simulink model "rosberrypi_publish_camera"  (R2018b)
settings: Solver=FixedStepAuto  StartTime=0.0  StopTime=inf  RelTol=1e-3  EnableMultiTasking=on
model workspace (MAT data in the model file):
  SL_ROS_VariableLengthArrays_MaxSizes.CommonInfo.ArrayTruncateAction = 'EmitWarning'
  SL_ROS_VariableLengthArrays_MaxSizes.MsgTypeMap = containers.Map
  SL_ROS_VariableLengthArrays_MaxSizes.MsgTypeMap.serialization.keys = {'sensor_msgs/Image'}
  SL_ROS_VariableLengthArrays_MaxSizes.MsgTypeMap.serialization.values{1}(1).PropertyName = 'Encoding'
  SL_ROS_VariableLengthArrays_MaxSizes.MsgTypeMap.serialization.values{1}(1).DataType = 'uint8'
  SL_ROS_VariableLengthArrays_MaxSizes.MsgTypeMap.serialization.values{1}(1).MaxLength = 5
  SL_ROS_VariableLengthArrays_MaxSizes.MsgTypeMap.serialization.values{1}(2).PropertyName = 'Data'
  SL_ROS_VariableLengthArrays_MaxSizes.MsgTypeMap.serialization.values{1}(2).DataType = 'uint8'
  SL_ROS_VariableLengthArrays_MaxSizes.MsgTypeMap.serialization.values{1}(2).MaxLength = 19200
  SL_ROS_VariableLengthArrays_MaxSizes.MsgTypeMap.serialization.uniformity = 0
  SL_ROS_VariableLengthArrays_MaxSizes.MsgTypeMap.serialization.keyType = 'char'
  SL_ROS_VariableLengthArrays_MaxSizes.MsgTypeMap.serialization.valueType = 'any'
libraries: robotlib x2, simulink x1, embdlinuxlib x1
settings Model: Creator=The MathWorks, Inc.  LastModifiedBy=The MathWorks, Inc.
settings DataIOCC: SaveFormat=Array
settings OptimizationCC: LifeSpan=Inf  MaxStackSize=64
settings DebuggingCC: SolverPrmCheckMsg=warning  AllowSymbolicDim=off  SFUnexpectedBacktrackingDiag=warning  SFNoUnconditionalDefaultTransitionDiag=warning  SFExecutionAtInitializationDiag=none
settings HardwareCC: ProdBitPerPointer=32  ProdBitPerSizeT=32  ProdBitPerPtrDiffT=32  ProdLargestAtomicInteger=Long  ProdLargestAtomicFloat=Double  ProdWordSize=32  ProdHWDeviceType=ARM Compatible->ARM Cortex
settings ModelReferenceCC: PropagateSignalLabelsOutOfModel=off
settings SFSimCC: SimUseLocalCustomCode=off  MATLABDynamicMemAlloc=off
settings RTWCC: SystemTargetFile=ert.tlc  HardwareBoard=Raspberry Pi - Robot Operating System (ROS)  TemplateMakefile=ert_default_tmf  GenerateReport=on  RTWUseLocalCustomCode=off  Toolchain=Catkin  IncludeHyperlinkInReport=on  LaunchReport=on  TargetLang=C++  GenerateTraceInfo=on  GenerateTraceReport=on  GenerateTraceReportSl=on  GenerateTraceReportSf=on  GenerateTraceReportEml=on
settings CodeAppCC: ForceParamTrailComments=on  OperatorAnnotations=on  SimulinkDataObjDesc=on  SFDataObjDesc=on  MATLABFcnDesc=on  InsertBlockDesc=on  StateflowObjectComments=on  MATLABSourceComments=on
settings ERTTargetCC: MultiwordLength=2048  MultiInstanceERTCode=on  CodeInterfacePackaging=C++ class  RootIOFormat=Structure reference
settings ConfigComp: CovMetricSettings=dw  CovHtmlReporting=on  CovSaveCumulativeToWorkspaceVar=on  CovSaveSingleToWorkspaceVar=on  CovExternalEMLEnable=off  CovSFcnEnable=off

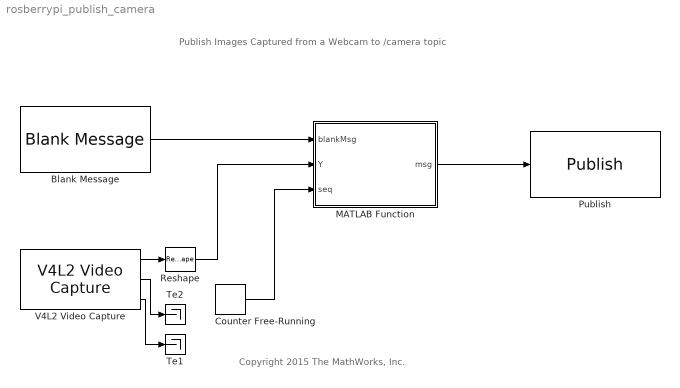
== system rosberrypi_publish_camera ==
  note: Publish Images Captured from
      | a Webcam to /camera topic
  note: Copyright 2015 The MathWorks, Inc.
  Blank Message : robotlib/Blank Message  messageType=sensor_msgs/Image  SampleTime=1/15
      settings: SourceProductBaseCode=RO
  Counter Free-Running : simulink/Sources/Counter Free-Running  NumBits=32  tsamp=-1
  MATLAB Function : MATLAB Function  TreatAsAtomicUnit=on
  Publish : robotlib/Publish  topicSource=Specify your own  topic=/camera  messageType=sensor_msgs/Image  messageQueueLength=1
      settings: SourceProductBaseCode=RO
  Reshape : Reshape
  Te1 : Terminator
  Te2 : Terminator
  V4L2 Video Capture : embdlinuxlib/V4L2 Video Capture  m_devName='/dev/video0'  roi=[0, 0, 640, 480]  imSizeSelection=160x120  imSize=[640, 480]  pixelFormat=YCbCr 4:2:2  pixelOrder=Planar  sampleTime=1/15  simOutput=Colorbars  blockPlatform=Raspberry Pi
      settings: SourceProductName=Simulink Support Package for Raspberry Pi Hardware  SourceProductBaseCode=RASPPI
  wires:
  V4L2 Video Capture/1 -> Reshape/1
  Reshape/1 -> MATLAB Function/2(Y)
  Counter Free-Running/1 -> MATLAB Function/3(seq)
  Blank Message/1 -> MATLAB Function/1(blankMsg)
  MATLAB Function/1(msg) -> Publish/1
  V4L2 Video Capture/2 -> Te2/1
  V4L2 Video Capture/3 -> Te1/1

== matlab function rosberrypi_publish_camera/MATLAB Function ==
  data: blankMsg input Bus: SL_Bus_rosberrypi_publish_camera_sensor_msgs_Image; msg output Bus: SL_Bus_rosberrypi_publish_camera_sensor_msgs_Image =0; Y input; seq input
function msg = fcn(blankMsg,Y,seq)
%#codegen

% To set datatype of MSG output:
%  1. Create buses for this model: robotics.ros.createSimulinkBus(gcs)
%  1. Click "Edit Data" in  Toolstrip to open "Ports and Data Manager"
%  2. Select MSG and set datatype to "Bus: SL_Bus_<modelname>_<messageType>"
% See: 
% http://www.mathworks.com/help/simulink/ug/create-structures-in-matlab-function-blocks.html

% blankMsg (sensor_msgs/Image) consists of 
%             Header: [1x1 Header]
%             uint32 Height
%             uint32 Width
%             string Encoding
%             uint8 Is_bigendian
%             uint32 Step
%             uint8[] Data


% Set width and height 
msg = blankMsg;
msg.Width = uint32(160);
msg.Height = uint32(120);

% Black and white image
msg.Encoding_SL_Info.CurrentLength = uint32(5);
msg.Encoding = uint8('mono8')';

% Size of image buffer = 160 * 120
msg.Data_SL_Info.CurrentLength = uint32(19200);
msg.Data = Y;

% Sequence number
msg.Header.Seq = seq;
end
